simulink model "ControlsWithAutopilot_Properties"  (Simulink 8.4)
settings: Solver=ode45  StartTime=0.0  StopTime=10.0  RelTol=1e-3
undefined symbols (not defined in the file): ap, bias
libraries: simulink x3, discretizing x1
(part 2 of 3)

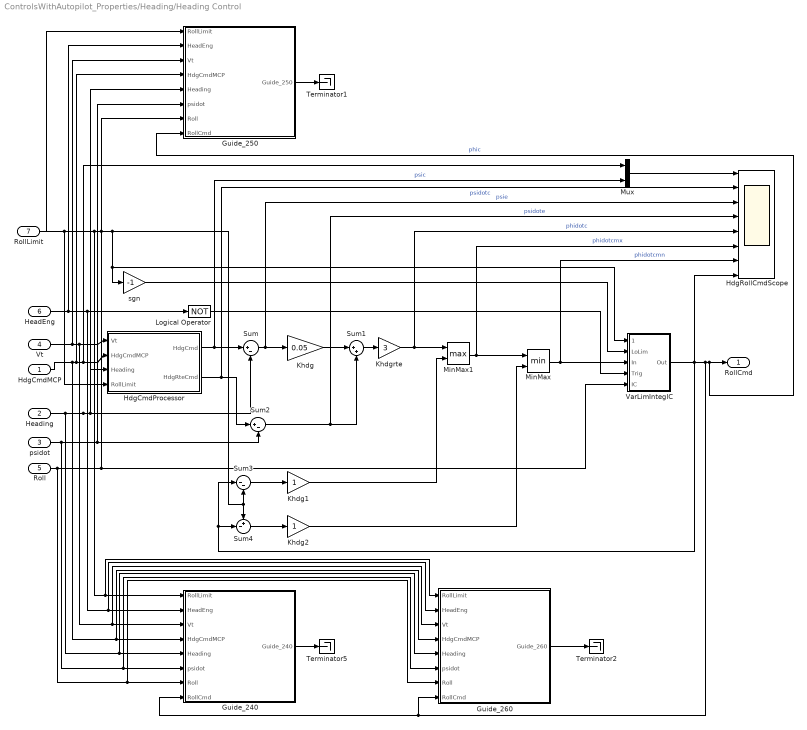
== system ControlsWithAutopilot_Properties/Heading/Heading Control ==
  HdgCmdMCP : Inport  RequirementInfo={} %GIDa_afcd05d1_a9dc_45a7_a8f8_7136ccc61726
  Heading : Inport  RequirementInfo={} %GIDa_19b80fe4_d265_482c_b709_18db80a7cdf3  Port=2
  psidot : Inport  RequirementInfo={} %GIDa_e421e82d_0cc7_4ad7_ac7a_9fb430d189d5  Port=3
  Vt : Inport  RequirementInfo={} %GIDa_9daf3e20_e00e_4f36_b534_d9747a241338  Port=4
  Roll : Inport  RequirementInfo={} %GIDa_8629ba77_a751_4097_af53_617eaa1017be  Port=5
  HeadEng : Inport  RequirementInfo={} %GIDa_dadb1310_2bf4_48cf_8970_85174d784ee3  Port=6
  RollLimit : Inport  Port=7
  Guide_240 : Subsystem  TreatAsAtomicUnit=on  mask(Observer){AnnotationType=ensures, ObserverType=ellipsoid}
      mask prompts: AnnotationType "Type of annotation (pre/post...)"; ObserverType "Observer type"
      mask help:
      | Set an observer for the system.
      | The annotation type parameter sets the type of observer:
      | - requires : pre-condition
      | - ensures : post-condition
      | - assert : an assertion
      | - observer : the observer computes a special type of properties
      mask TypeOptions AnnotationType: ensures | requires | assert | observer
      mask Callback AnnotationType:
      | paramStr = get_param(gcb, 'MaskValues');
      | 
      | if strcmp(paramStr{1}(1),'o')
      |     set_param(gcb,'MaskVisibilities',{'on';'on'});
      |     paramStr{2} = 'ellipsoid';
      |     set_param(gcb,'MaskValues',paramStr);
      | else
      |     set_param(gcb,'MaskVisibilities',{'on';'off'});
      | end
      mask Callback ObserverType:
      | paramStr = get_param(gcb, 'MaskValues');
      | 
      | if strcmp(paramStr{1}(1),'observer')
      |     set_param(gcb,'MaskVisibilities',{'on';'on'});
      |     paramStr{2} = 'ellipsoid';
      |     set_param(gcb,'MaskValues',paramStr);
      | else
      |     set_param(gcb,'MaskVisibilities',{'on';'off'});
      | end
      mask Display:
      | color('red');
      | text(0.5, 0.5, 'Observer Block', 'horizontalAlignment', 'center');
  Guide_250 : Subsystem  TreatAsAtomicUnit=on  mask(Observer){AnnotationType=ensures, ObserverType=ellipsoid}
      mask prompts: AnnotationType "Type of annotation (pre/post...)"; ObserverType "Observer type"
      mask help:
      | Set an observer for the system.
      | The annotation type parameter sets the type of observer:
      | - requires : pre-condition
      | - ensures : post-condition
      | - assert : an assertion
      | - observer : the observer computes a special type of properties
      mask TypeOptions AnnotationType: ensures | requires | assert | observer
      mask Callback AnnotationType:
      | paramStr = get_param(gcb, 'MaskValues');
      | 
      | if strcmp(paramStr{1}(1),'o')
      |     set_param(gcb,'MaskVisibilities',{'on';'on'});
      |     paramStr{2} = 'ellipsoid';
      |     set_param(gcb,'MaskValues',paramStr);
      | else
      |     set_param(gcb,'MaskVisibilities',{'on';'off'});
      | end
      mask Callback ObserverType:
      | paramStr = get_param(gcb, 'MaskValues');
      | 
      | if strcmp(paramStr{1}(1),'observer')
      |     set_param(gcb,'MaskVisibilities',{'on';'on'});
      |     paramStr{2} = 'ellipsoid';
      |     set_param(gcb,'MaskValues',paramStr);
      | else
      |     set_param(gcb,'MaskVisibilities',{'on';'off'});
      | end
      mask Display:
      | color('red');
      | text(0.5, 0.5, 'Observer Block', 'horizontalAlignment', 'center');
  Guide_260 : Subsystem  TreatAsAtomicUnit=on  mask(Observer){AnnotationType=ensures, ObserverType=ellipsoid}
      mask prompts: AnnotationType "Type of annotation (pre/post...)"; ObserverType "Observer type"
      mask help:
      | Set an observer for the system.
      | The annotation type parameter sets the type of observer:
      | - requires : pre-condition
      | - ensures : post-condition
      | - assert : an assertion
      | - observer : the observer computes a special type of properties
      mask TypeOptions AnnotationType: ensures | requires | assert | observer
      mask Callback AnnotationType:
      | paramStr = get_param(gcb, 'MaskValues');
      | 
      | if strcmp(paramStr{1}(1),'o')
      |     set_param(gcb,'MaskVisibilities',{'on';'on'});
      |     paramStr{2} = 'ellipsoid';
      |     set_param(gcb,'MaskValues',paramStr);
      | else
      |     set_param(gcb,'MaskVisibilities',{'on';'off'});
      | end
      mask Callback ObserverType:
      | paramStr = get_param(gcb, 'MaskValues');
      | 
      | if strcmp(paramStr{1}(1),'observer')
      |     set_param(gcb,'MaskVisibilities',{'on';'on'});
      |     paramStr{2} = 'ellipsoid';
      |     set_param(gcb,'MaskValues',paramStr);
      | else
      |     set_param(gcb,'MaskVisibilities',{'on';'off'});
      | end
      mask Display:
      | color('red');
      | text(0.5, 0.5, 'Observer Block', 'horizontalAlignment', 'center');
  HdgCmdProcessor : Subsystem  RequirementInfo={} %GIDa_3cb77e5f_f630_4f22_88a8_7528bfceb83f
  HdgRollCmdScope : Scope  NumInputPorts=8
      settings: RequirementInfo={} %GIDa_5fbe2135_fdf1_4f64_a179_faa1710ae21e  YMin=-30~-30~-10~-10~-4~-10~0~-5  YMax=30~30~10~10~4~10~1~5  SaveName=ScopeData7
  Khdg : Gain  RequirementInfo={} %GIDa_abf81b08_c210_4343_b4da_5a7e229caeb6  Gain=0.05
  Khdg1 : Gain  RequirementInfo={} %GIDa_7a7a35ca_24a5_4d20_bc30_55deea16462c
  Khdg2 : Gain  RequirementInfo={} %GIDa_57191899_7ee5_4454_897a_7009651ed5fb
  Khdgrte : Gain  RequirementInfo={} %GIDa_bcc6a420_18f3_43f0_aaa1_aaa1bbf90f64  Gain=3
  Logical Operator : Logic  RequirementInfo={} %GIDa_5ad405ac_0a88_4b96_aa0e_75483351ee25  Operator=NOT  AllPortsSameDT=off  OutDataTypeStr=boolean
  MinMax : MinMax  RequirementInfo={} %GIDa_4b9381d8_eb85_418b_a975_85846d5ca8c2  Inputs=2
  MinMax1 : MinMax  RequirementInfo={} %GIDa_b40e082d_0fb2_4088_baf4_e9a71be9bcc1  Function=max  Inputs=2
  Mux : Mux  RequirementInfo={} %GIDa_0e83f6c6_ae04_43dd_95fe_a79ec32b40e2  Inputs=2
  Sum : Sum  RequirementInfo={} %GIDa_b89885fc_f86c_4a50_8ce5_47d0488bdc1c  Inputs=|+-
  Sum1 : Sum  RequirementInfo={} %GIDa_40ec6862_b1f8_4f97_ae14_1eadabbceb30  Inputs=|++
  Sum2 : Sum  RequirementInfo={} %GIDa_307d6880_3ab8_4deb_90e0_d68f11d87c85  Inputs=|+-
  Sum3 : Sum  RequirementInfo={} %GIDa_ebb8b765_7f4a_435f_be61_680d3199141b  Inputs=|--
  Sum4 : Sum  RequirementInfo={} %GIDa_05638559_562a_476e_9e4c_91124434a43b  Inputs=+-|
  Terminator1 : Terminator
  Terminator2 : Terminator
  Terminator5 : Terminator
  VarLimIntegIC : Subsystem  RequirementInfo={} %GIDa_7da7eaf5_9731_498e_9aad_b41279918004
  sgn : Gain  RequirementInfo={} %GIDa_84e2dc00_f2e5_41f4_89ce_c9fef234974f  Gain=-1
  RollCmd : Outport  RequirementInfo={} %GIDa_aa862f7f_5d4e_408f_b8c4_26b4ce96fbda
  wires:
  Heading/1 -> Sum/2, HdgCmdProcessor/3(Heading), Guide_250/5(Heading), Guide_240/5(Heading), Guide_260/5(Heading)
  HdgCmdProcessor/1(HdgCmd) -> Sum/1, Mux/2  "psic"
  Sum/1 -> Khdg/1, HdgRollCmdScope/3  "psie"
  Khdg/1 -> Sum1/1
  Sum2/1 -> Sum1/2, HdgRollCmdScope/4  "psidote"
  HdgCmdProcessor/2(HdgRteCmd) -> Sum2/1, HdgRollCmdScope/2  "psidotc"
  psidot/1 -> Sum2/2, Guide_250/6(psidot), Guide_240/6(psidot), Guide_260/6(psidot)
  Vt/1 -> HdgCmdProcessor/1(Vt), Guide_240/3(Vt), Guide_260/3(Vt), Guide_250/3(Vt)
  HdgCmdMCP/1 -> HdgCmdProcessor/2(HdgCmdMCP), Mux/1, Guide_250/4(HdgCmdMCP), Guide_240/4(HdgCmdMCP), Guide_260/4(HdgCmdMCP)
  VarLimIntegIC/1(Out) -> Sum3/1, Sum4/2, HdgRollCmdScope/8, RollCmd/1, Guide_250/8(RollCmd), Guide_240/8(RollCmd), Guide_260/8(RollCmd)  "phic"
  RollLimit/1 -> HdgCmdProcessor/4(RollLimit), Sum4/1, Sum3/2, VarLimIntegIC/1(UpLim), sgn/1, Guide_250/1(RollLimit), Guide_240/1(RollLimit), Guide_260/1(RollLimit)
  sgn/1 -> VarLimIntegIC/2(LoLim)
  Sum1/1 -> Khdgrte/1
  MinMax1/1 -> MinMax/1, HdgRollCmdScope/6  "phidotcmx"
  MinMax/1 -> VarLimIntegIC/3(In), HdgRollCmdScope/7  "phidotcmn"
  HeadEng/1 -> Logical Operator/1, Guide_240/2(HeadEng), Guide_260/2(HeadEng), Guide_250/2(HeadEng)
  Sum3/1 -> Khdg1/1
  Sum4/1 -> Khdg2/1
  Khdg1/1 -> MinMax1/2
  Khdg2/1 -> MinMax/2
  Roll/1 -> VarLimIntegIC/5(IC), Guide_250/7(Roll), Guide_240/7(Roll), Guide_260/7(Roll)
  Khdgrte/1 -> MinMax1/1, HdgRollCmdScope/5  "phidotc"
  Logical Operator/1 -> VarLimIntegIC/4(Trig)
  Mux/1 -> HdgRollCmdScope/1
  Guide_240/1(Guide_240) -> Terminator5/1
  Guide_250/1(Guide_250) -> Terminator1/1
  Guide_260/1(Guide_260) -> Terminator2/1

== system ControlsWithAutopilot_Properties/Heading/ManualOverride ==
  Man : Inport
  Auto : Inport  Port=2
  Switch1 : Switch  RequirementInfo={} %GIDa_5800ea93_45af_42da_974c_4cd975d0b8c8  Criteria=u2 ~= 0  Threshold=0.5
  Out : Outport
  wires:
  Man/1 -> Switch1/3, Switch1/2
  Auto/1 -> Switch1/1
  Switch1/1 -> Out/1

== system ControlsWithAutopilot_Properties/Heading/Roll InnerLoop ==
  note: orig =[0 60 140]
  note: orig = 0.25
  note: orig = 0.8
  RollCmd : Inport  RequirementInfo={} %GIDa_549f9d91_ca5c_4ec7_bf56_cf05f3793396
  Roll : Inport  RequirementInfo={} %GIDa_d885705c_af8c_4e18_b4d1_2f073687ea2c  Port=2
  pdeg : Inport  RequirementInfo={} %GIDa_ba7aa095_15b8_4f85_9051_8b947d28a24d  Port=3
  CAS : Inport  RequirementInfo={} %GIDa_defe4f55_1722_479a_b684_dc07a497c4ef  Port=4
  Kcas_pp : Subsystem  TreatAsAtomicUnit=on
  Kphierr : Gain  RequirementInfo={} %GIDa_96c602a9_a07d_4519_9a2c_04c20a8c958d  Gain=0.5
  Product : Product  RequirementInfo={} %GIDa_6029a1e1_bbec_4e58_a2a6_3f9df62d6e90  RndMeth=Zero
  Roll_IL_scope : Scope  NumInputPorts=7
      settings: RequirementInfo={} %GIDa_ec5ee575_c049_4397_a5dd_5347629f97a6  YMin=-30~-30~-10~-10~-4~-10~0  YMax=30~30~10~10~4~10~1  SaveName=ScopeData5
  Sum : Sum  RequirementInfo={} %GIDa_6dd565f9_cc9c_463a_985b_c182e040d7fd  Inputs=|+-
  Sum1 : Sum  RequirementInfo={} %GIDa_02561aa6_0360_4e6c_b76e_5dde7f2ab3b1  Inputs=|+-
  rollrate_IL : discretizing/Discretized Zero-Pole  RequirementInfo={} %GIDa_636569be_bc7e_4244_84a4_4a62b7fc0808  Zeros=0  Poles=-0.5  Gain=0.00645  AbsTol=auto  SampleTime=1.0  method=zoh  Wc=1
  AilCmd : Outport  RequirementInfo={} %GIDa_cd7ddcd8_c7c7_43e2_be4e_2c0bb3f4c702
  wires:
  Product/1 -> AilCmd/1, Roll_IL_scope/6  "ailcmd"
  Kcas_pp/1(Out) -> Product/2, Roll_IL_scope/7  "kcas"
  Sum1/1 -> Product/1
  CAS/1 -> Kcas_pp/1(In)
  rollrate_IL/1 -> Sum1/2, Roll_IL_scope/5  "pdegwo"
  pdeg/1 -> rollrate_IL/1, Roll_IL_scope/4  "pdeg"
  Kphierr/1 -> Sum1/1
  Roll/1 -> Sum/2, Roll_IL_scope/2  "roll"
  Sum/1 -> Kphierr/1, Roll_IL_scope/3  "rollerr"
  RollCmd/1 -> Sum/1, Roll_IL_scope/1  "rollcmd"

== system ControlsWithAutopilot_Properties/Longitudinal/Altitude Control ==
  engage : Inport  RequirementInfo={} %GIDa_92edc9e2_4cfd_4b16_8fee_8b94964575da
  AltCmd : Inport  RequirementInfo={} %GIDa_edbc7e5c_23e1_4d8f_98c5_e2d77895a510  Port=2
  Altitude : Inport  RequirementInfo={} %GIDa_01b40abf_ece8_4194_aeed_7639b2f9d320  Port=3
  gskts : Inport  RequirementInfo={} %GIDa_49aaf918_ec6b_4cc9_bdad_efb02f39ea3b  Port=4
  hdot : Inport  RequirementInfo={} %GIDa_f8353919_6ca2_40ed_9884_9c34b61b1365  Port=5
  hdotChgRate : Inport  Port=6
  maxHdotChg : Inport  Port=7
  Abs : Abs  RequirementInfo={} %GIDa_1391aa7c_5846_4be5_914e_111d8f2c4215  SaturateOnIntegerOverflow=on
  AltCtnlScope : Scope  NumInputPorts=3
      settings: RequirementInfo={} %GIDa_baad481c_a27b_41ac_bf32_d6e1a7f2cfe1  TimeRange=30  YMin=10000~-5~0  YMax=10200~15~1  SaveName=ScopeData3
  Constant1 : Constant  RequirementInfo={} %GIDa_566c4b52_316f_4d36_82bb_fb65e53f78d2  Value=0
  Divide : Product  RequirementInfo={} %GIDa_b9d1a3fe_7e00_46b2_9426_cf952dcaf391  Inputs=*/
  Kh : Gain  RequirementInfo={} %GIDa_de6b2d53_b3f4_42e2_83e9_439be9ccc299  Gain=0.08
  Logical Operator : Logic  RequirementInfo={} %GIDa_921e6188_0ac2_4a9c_befc_5c7a6835e9e6  Operator=NOT
  Mux : Mux  RequirementInfo={} %GIDa_68aa779e_2c07_4c3b_9ca1_0ecb3161e49a  Inputs=2
  Mux1 : Mux  RequirementInfo={} %GIDa_0a0909f8_d09a_4568_9828_3f29982a74b3  Inputs=2
  Saturation : Saturate  RequirementInfo={} %GIDa_77166b67_e163_40e1_b7e4_7e7410a56d29  UpperLimit=1000  LowerLimit=0.0001
  Sum : Sum  RequirementInfo={} %GIDa_d94a0856_9d8d_4fca_8b77_5f1cf21c0c3a  Inputs=|+-
  Sum3 : Sum  RequirementInfo={} %GIDa_3ee7802b_411f_4586_886f_8bdef6cfccb9  Inputs=|++  SaturateOnIntegerOverflow=on  InputSameDT=on  OutDataTypeStr=Inherit: Same as first input
  Switch : Switch  RequirementInfo={} %GIDa_64af29d5_be60_4de8_bcf5_833ab8e70f35
  Variable  Rate Limit : Subsystem  RequirementInfo={} %GIDa_7d0e1926_4469_4591_916e_2bb88ddee008  TreatAsAtomicUnit=on
  Variable Limit Saturation : Subsystem  RequirementInfo={} %GIDa_0b931211_59c1_4508_94b8_12d4cca2cb6b  TreatAsAtomicUnit=on
  k : Gain  RequirementInfo={} %GIDa_65a0c0b6_6e9b_4a97_b326_1d79079cc625  Gain=-1
  kts2fps : Gain  RequirementInfo={} %GIDa_a49848e7_9841_44de_8ec7_08f1ed28d1e0  Gain=1.6878
  r2d : Gain  RequirementInfo={} %GIDa_934ba914_aaac_471d_9b5e_a120031a3853  Gain=57.2958
  altgamcmd : Outport  RequirementInfo={} %GIDa_3c331913_004d_4e8f_a0a1_b052c80c7670
  wires:
  Sum/1 -> Kh/1
  AltCmd/1 -> Sum/1, Mux/1  "AltCmd"
  Altitude/1 -> Sum/2, Mux/2  "Alt"
  hdot/1 -> Abs/1, Variable  Rate Limit/4(IC)
  Abs/1 -> Sum3/1
  maxHdotChg/1 -> Sum3/2
  k/1 -> Variable Limit Saturation/3(Lo_lim)
  Sum3/1 -> k/1, Variable Limit Saturation/1(up_lim)
  engage/1 -> Switch/2, Logical Operator/1, AltCtnlScope/3  "alteng"
  gskts/1 -> kts2fps/1
  Divide/1 -> r2d/1
  r2d/1 -> altgamcmd/1
  Logical Operator/1 -> Variable  Rate Limit/3(ICtrig)
  Variable Limit Saturation/1(Out1) -> Variable  Rate Limit/2(input), Mux1/1  "hdotc"
  hdotChgRate/1 -> Variable  Rate Limit/1(ratelim)
  Variable  Rate Limit/1(output) -> Divide/1, Mux1/2  "hdotcLim"
  kts2fps/1 -> Saturation/1
  Saturation/1 -> Divide/2
  Switch/1 -> Variable Limit Saturation/2(SigIn)
  Kh/1 -> Switch/1
  Constant1/1 -> Switch/3
  Mux/1 -> AltCtnlScope/1
  Mux1/1 -> AltCtnlScope/2

== system ControlsWithAutopilot_Properties/Longitudinal/EngageORzero ==
  Engage : Inport
  In : Inport  Port=2
  Logical Operator5 : Logic  RequirementInfo={} %GIDa_2faaa958_fdd5_4161_8224_87bc655595ec  AllPortsSameDT=off  OutDataTypeStr=boolean
  Switch1 : Switch  RequirementInfo={} %GIDa_cd8505b1_f38c_41a3_a83c_5e083797b181  Threshold=0.5
  zero10 : Constant  RequirementInfo={} %GIDa_596a5899_ba53_4c37_8272_7211e27ddf24
  zero9 : Constant  RequirementInfo={} %GIDa_b5c8c028_3d9d_45c0_afd9_41cf87627ef7  Value=0
  Out : Outport
  wires:
  Engage/1 -> Logical Operator5/1
  zero10/1 -> Logical Operator5/2
  zero9/1 -> Switch1/3
  In/1 -> Switch1/1
  Logical Operator5/1 -> Switch1/2
  Switch1/1 -> Out/1

== system ControlsWithAutopilot_Properties/Longitudinal/FPA Control ==
  engage : Inport  RequirementInfo={} %GIDa_4330a6b4_8fd7_4be4_8132_0a5a51cb5321
  gamcmd : Inport  RequirementInfo={} %GIDa_72bd14a4_cf4e_4ddf_9979_bc189fd4e864  Port=2
  gamma : Inport  RequirementInfo={} %GIDa_07a290a4_e9be_4e9c_ae2b_d72f5ca4cb2b  Port=3
  thetadeg : Inport  RequirementInfo={} %GIDa_6ddd8d11_1197_4928_a2bc_231a82446ee7  Port=4
  VT : Inport  RequirementInfo={} %GIDa_a0a43ff9_fad6_4fc8_a8cd_c357b3dfb673  Port=5
  FPAScope : Scope  NumInputPorts=4
      settings: RequirementInfo={} %GIDa_08c55925_5efe_4d90_b09d_0072cafa98d7  YMin=-1~-5~-2~-5  YMax=2~5~2~10  SaveName=ScopeData12
  Integ_FPA : DiscreteIntegrator  ExternalReset=level  InitialConditionSource=external  SampleTime=1.0  mask(DiscretizedDiscreteIntegrator){}
      mask init:
      | %zoh
  KIgamerr : Gain  RequirementInfo={} %GIDa_08963e9e_c311_47c8_a63e_11cc7c9fb2d8
  Kgamerr : Gain  RequirementInfo={} %GIDa_3495b1a6_277d_4a6c_aa4f_649fc83b9092  Gain=1.4
  Logical Operator : Logic  RequirementInfo={} %GIDa_eba75fd0_479d_4894_b4e0_0ecea241815c  Operator=NOT  AllPortsSameDT=off  OutDataTypeStr=boolean
  Mux : Mux  RequirementInfo={} %GIDa_ae1e9d70_29ff_4004_97f5_396f2626ff0e  Inputs=2
  Mux1 : Mux  RequirementInfo={} %GIDa_b657458f_9c9c_48b1_af95_f550cfeae5f6  Inputs=2
  Product1 : Product  RequirementInfo={} %GIDa_bb863780_5e58_4e21_8791_e7a2c94dd786  RndMeth=Zero
  Saturation Dynamic : simulink/Discontinuities/Saturation Dynamic  OutMin=[]  OutMax=[]  OutDataTypeStr=Inherit: Same as second input  OutDataType=fixdt(1, 16)  OutScaling=2^-10  DoSatur=off
  Sum : Sum  RequirementInfo={} %GIDa_494c7255_4427_4dad_a3c1_4aee399936eb  Inputs=|++
  Sum1 : Sum  RequirementInfo={} %GIDa_93359946_60e9_438e_99e8_9beddee58b77  Inputs=|+-
  Sum2 : Sum  RequirementInfo={} %GIDa_c5e9feb7_f19d_4066_9b64_2fe045a465c2  Inputs=|+-
  hddLim : Constant  RequirementInfo={} %GIDa_1bf124ef_f3a0_4770_a704_52ef6436d4b5  Value=4.83*57.2958
  kt2fps : Gain  RequirementInfo={} %GIDa_c7ee5a6f_140d_48a3_b5c5_8ced7bef0603  Gain=1.6878
  m1 : Gain  RequirementInfo={} %GIDa_3e310fb8_58d1_4ad2_a1bc_b1914379a108  Gain=-1
  PitchCmd : Outport  RequirementInfo={} %GIDa_7e56bb7b_bd21_4466_8889_6a6d9858a2da
  wires:
  Sum1/1 -> PitchCmd/1, FPAScope/4  "PitchCmd"
  Kgamerr/1 -> Sum1/2, Sum/2
  Integ_FPA/1 -> Sum1/1
  gamma/1 -> Kgamerr/1, Sum2/2, Mux/2  "gamma"
  thetadeg/1 -> Sum/1
  Sum/1 -> Integ_FPA/3
  engage/1 -> Logical Operator/1, FPAScope/1  "engage"
  Logical Operator/1 -> Integ_FPA/2
  kt2fps/1 -> Product1/2
  hddLim/1 -> Product1/1
  Product1/1 -> Saturation Dynamic/1, m1/1
  VT/1 -> kt2fps/1
  Saturation Dynamic/1 -> Integ_FPA/1, Mux1/2  "gamerrlim"
  KIgamerr/1 -> Saturation Dynamic/2
  m1/1 -> Saturation Dynamic/3
  Sum2/1 -> KIgamerr/1, Mux1/1  "gamerr"
  gamcmd/1 -> Sum2/1, Mux/1  "gamcmd"
  Mux/1 -> FPAScope/2
  Mux1/1 -> FPAScope/3

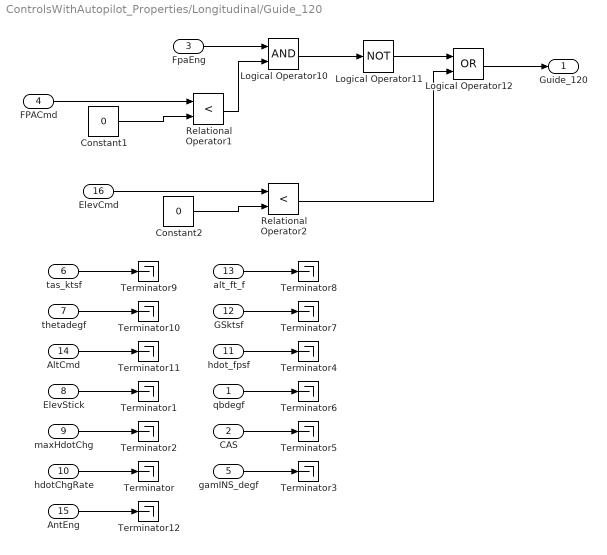
== system ControlsWithAutopilot_Properties/Longitudinal/Guide_120 ==
  qbdegf : Inport
  CAS : Inport  Port=2
  FpaEng : Inport  Port=3
  FPACmd : Inport  Port=4
  gamINS_degf : Inport  Port=5
  tas_ktsf : Inport  Port=6
  thetadegf : Inport  Port=7
  ElevStick : Inport  Port=8
  maxHdotChg : Inport  Port=9
  hdotChgRate : Inport  Port=10
  hdot_fpsf : Inport  Port=11
  GSktsf : Inport  Port=12
  alt_ft_f : Inport  Port=13
  AltCmd : Inport  Port=14
  AntEng : Inport  Port=15
  ElevCmd : Inport  Port=16
  Constant1 : Constant  Value=0
  Constant2 : Constant  Value=0
  Logical Operator10 : Logic  AllPortsSameDT=off  OutDataTypeStr=boolean
  Logical Operator11 : Logic  Operator=NOT  AllPortsSameDT=off  OutDataTypeStr=boolean
  Logical Operator12 : Logic  Operator=OR  AllPortsSameDT=off  OutDataTypeStr=boolean
  Relational Operator1 : RelationalOperator  Operator=<  OutDataTypeStr=boolean
  Relational Operator2 : RelationalOperator  Operator=<  OutDataTypeStr=boolean
  Terminator{,1..12} (13 alike) : Terminator
  Guide_120 : Outport
  wires:
  hdotChgRate/1 -> Terminator/1
  maxHdotChg/1 -> Terminator2/1
  ElevStick/1 -> Terminator1/1
  CAS/1 -> Terminator5/1
  qbdegf/1 -> Terminator6/1
  Constant2/1 -> Relational Operator2/2
  ElevCmd/1 -> Relational Operator2/1
  FpaEng/1 -> Logical Operator10/1
  Constant1/1 -> Relational Operator1/2
  FPACmd/1 -> Relational Operator1/1
  Relational Operator1/1 -> Logical Operator10/2
  Logical Operator11/1 -> Logical Operator12/1
  Logical Operator10/1 -> Logical Operator11/1
  Relational Operator2/1 -> Logical Operator12/2
  Logical Operator12/1 -> Guide_120/1
  alt_ft_f/1 -> Terminator8/1
  GSktsf/1 -> Terminator7/1
  hdot_fpsf/1 -> Terminator4/1
  gamINS_degf/1 -> Terminator3/1
  tas_ktsf/1 -> Terminator9/1
  thetadegf/1 -> Terminator10/1
  AltCmd/1 -> Terminator11/1
  AntEng/1 -> Terminator12/1

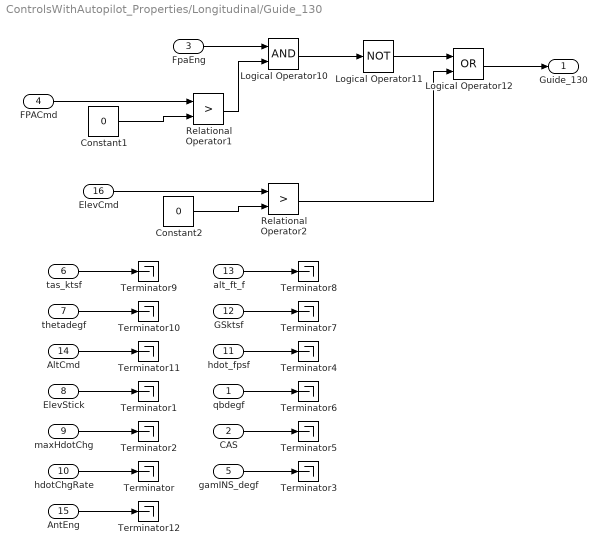
== system ControlsWithAutopilot_Properties/Longitudinal/Guide_130 ==
  qbdegf : Inport
  CAS : Inport  Port=2
  FpaEng : Inport  Port=3
  FPACmd : Inport  Port=4
  gamINS_degf : Inport  Port=5
  tas_ktsf : Inport  Port=6
  thetadegf : Inport  Port=7
  ElevStick : Inport  Port=8
  maxHdotChg : Inport  Port=9
  hdotChgRate : Inport  Port=10
  hdot_fpsf : Inport  Port=11
  GSktsf : Inport  Port=12
  alt_ft_f : Inport  Port=13
  AltCmd : Inport  Port=14
  AntEng : Inport  Port=15
  ElevCmd : Inport  Port=16
  Constant1 : Constant  Value=0
  Constant2 : Constant  Value=0
  Logical Operator10 : Logic  AllPortsSameDT=off  OutDataTypeStr=boolean
  Logical Operator11 : Logic  Operator=NOT  AllPortsSameDT=off  OutDataTypeStr=boolean
  Logical Operator12 : Logic  Operator=OR  AllPortsSameDT=off  OutDataTypeStr=boolean
  Relational Operator1 : RelationalOperator  Operator=>  OutDataTypeStr=boolean
  Relational Operator2 : RelationalOperator  Operator=>  OutDataTypeStr=boolean
  Terminator{,1..12} (13 alike) : Terminator
  Guide_130 : Outport
  wires:
  hdotChgRate/1 -> Terminator/1
  maxHdotChg/1 -> Terminator2/1
  ElevStick/1 -> Terminator1/1
  CAS/1 -> Terminator5/1
  qbdegf/1 -> Terminator6/1
  Constant2/1 -> Relational Operator2/2
  ElevCmd/1 -> Relational Operator2/1
  FpaEng/1 -> Logical Operator10/1
  Constant1/1 -> Relational Operator1/2
  FPACmd/1 -> Relational Operator1/1
  Relational Operator1/1 -> Logical Operator10/2
  Logical Operator11/1 -> Logical Operator12/1
  Logical Operator10/1 -> Logical Operator11/1
  Relational Operator2/1 -> Logical Operator12/2
  Logical Operator12/1 -> Guide_130/1
  alt_ft_f/1 -> Terminator8/1
  GSktsf/1 -> Terminator7/1
  hdot_fpsf/1 -> Terminator4/1
  gamINS_degf/1 -> Terminator3/1
  tas_ktsf/1 -> Terminator9/1
  thetadegf/1 -> Terminator10/1
  AltCmd/1 -> Terminator11/1
  AntEng/1 -> Terminator12/1

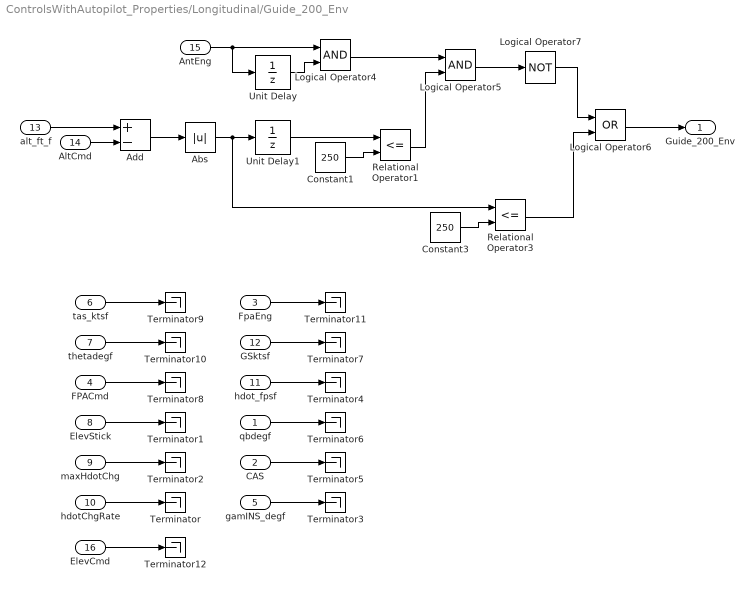
== system ControlsWithAutopilot_Properties/Longitudinal/Guide_200_Env ==
  qbdegf : Inport
  CAS : Inport  Port=2
  FpaEng : Inport  Port=3
  FPACmd : Inport  Port=4
  gamINS_degf : Inport  Port=5
  tas_ktsf : Inport  Port=6
  thetadegf : Inport  Port=7
  ElevStick : Inport  Port=8
  maxHdotChg : Inport  Port=9
  hdotChgRate : Inport  Port=10
  hdot_fpsf : Inport  Port=11
  GSktsf : Inport  Port=12
  alt_ft_f : Inport  Port=13
  AltCmd : Inport  Port=14
  AntEng : Inport  Port=15
  ElevCmd : Inport  Port=16
  Abs : Abs
  Add : Sum  Inputs=+-
  Constant1 : Constant  Value=250
  Constant3 : Constant  Value=250
  Logical Operator4 : Logic  AllPortsSameDT=off  OutDataTypeStr=boolean
  Logical Operator5 : Logic  AllPortsSameDT=off  OutDataTypeStr=boolean
  Logical Operator6 : Logic  Operator=OR  AllPortsSameDT=off  OutDataTypeStr=boolean
  Logical Operator7 : Logic  Operator=NOT  AllPortsSameDT=off  OutDataTypeStr=boolean
  Relational Operator1 : RelationalOperator  Operator=<=  OutDataTypeStr=boolean
  Relational Operator3 : RelationalOperator  Operator=<=  OutDataTypeStr=boolean
  Terminator{,1..12} (13 alike) : Terminator
  Unit Delay : UnitDelay  SampleTime=-1
  Unit Delay1 : UnitDelay  SampleTime=-1
  Guide_200_Env : Outport
  wires:
  hdotChgRate/1 -> Terminator/1
  maxHdotChg/1 -> Terminator2/1
  ElevStick/1 -> Terminator1/1
  CAS/1 -> Terminator5/1
  qbdegf/1 -> Terminator6/1
  GSktsf/1 -> Terminator7/1
  hdot_fpsf/1 -> Terminator4/1
  gamINS_degf/1 -> Terminator3/1
  tas_ktsf/1 -> Terminator9/1
  thetadegf/1 -> Terminator10/1
  FpaEng/1 -> Terminator11/1
  FPACmd/1 -> Terminator8/1
  ElevCmd/1 -> Terminator12/1
  AntEng/1 -> Unit Delay/1, Logical Operator4/1
  Unit Delay/1 -> Logical Operator4/2
  Logical Operator4/1 -> Logical Operator5/1
  Add/1 -> Abs/1
  AltCmd/1 -> Add/2
  alt_ft_f/1 -> Add/1
  Abs/1 -> Relational Operator3/1, Unit Delay1/1
  Constant1/1 -> Relational Operator1/2
  Unit Delay1/1 -> Relational Operator1/1
  Relational Operator1/1 -> Logical Operator5/2
  Logical Operator7/1 -> Logical Operator6/1
  Logical Operator5/1 -> Logical Operator7/1
  Constant3/1 -> Relational Operator3/2
  Relational Operator3/1 -> Logical Operator6/2
  Logical Operator6/1 -> Guide_200_Env/1

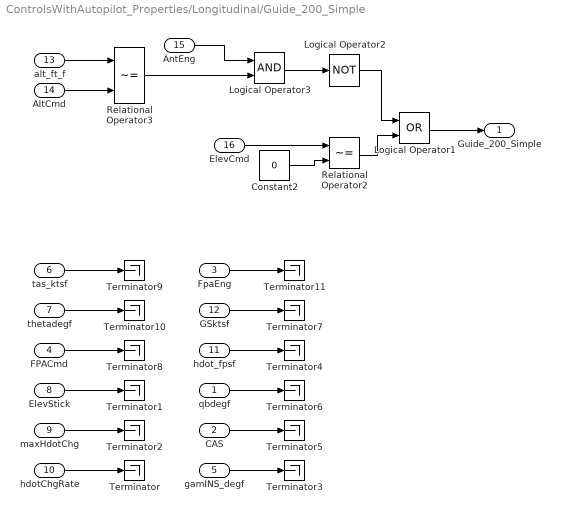
== system ControlsWithAutopilot_Properties/Longitudinal/Guide_200_Simple ==
  qbdegf : Inport
  CAS : Inport  Port=2
  FpaEng : Inport  Port=3
  FPACmd : Inport  Port=4
  gamINS_degf : Inport  Port=5
  tas_ktsf : Inport  Port=6
  thetadegf : Inport  Port=7
  ElevStick : Inport  Port=8
  maxHdotChg : Inport  Port=9
  hdotChgRate : Inport  Port=10
  hdot_fpsf : Inport  Port=11
  GSktsf : Inport  Port=12
  alt_ft_f : Inport  Port=13
  AltCmd : Inport  Port=14
  AntEng : Inport  Port=15
  ElevCmd : Inport  Port=16
  Constant2 : Constant  Value=0
  Logical Operator1 : Logic  Operator=OR  AllPortsSameDT=off  OutDataTypeStr=boolean
  Logical Operator2 : Logic  Operator=NOT  AllPortsSameDT=off  OutDataTypeStr=boolean
  Logical Operator3 : Logic  AllPortsSameDT=off  OutDataTypeStr=boolean
  Relational Operator2 : RelationalOperator  Operator=~=  OutDataTypeStr=boolean
  Relational Operator3 : RelationalOperator  Operator=~=  OutDataTypeStr=boolean
  Terminator{,1..11} (12 alike) : Terminator
  Guide_200_Simple : Outport
  wires:
  hdotChgRate/1 -> Terminator/1
  maxHdotChg/1 -> Terminator2/1
  ElevStick/1 -> Terminator1/1
  CAS/1 -> Terminator5/1
  qbdegf/1 -> Terminator6/1
  GSktsf/1 -> Terminator7/1
  hdot_fpsf/1 -> Terminator4/1
  gamINS_degf/1 -> Terminator3/1
  tas_ktsf/1 -> Terminator9/1
  thetadegf/1 -> Terminator10/1
  Constant2/1 -> Relational Operator2/2
  ElevCmd/1 -> Relational Operator2/1
  Relational Operator2/1 -> Logical Operator1/2
  Logical Operator2/1 -> Logical Operator1/1
  Logical Operator1/1 -> Guide_200_Simple/1
  AntEng/1 -> Logical Operator3/1
  alt_ft_f/1 -> Relational Operator3/1
  AltCmd/1 -> Relational Operator3/2
  Relational Operator3/1 -> Logical Operator3/2
  Logical Operator3/1 -> Logical Operator2/1
  FpaEng/1 -> Terminator11/1
  FPACmd/1 -> Terminator8/1

== system ControlsWithAutopilot_Properties/Longitudinal/ManualOverride ==
  Man : Inport
  Auto : Inport  Port=2
  Switch1 : Switch  RequirementInfo={} %GIDa_891c72b6_c029_43c0_848a_219761f8f015  Criteria=u2 ~= 0  Threshold=0.5
  Out : Outport
  wires:
  Man/1 -> Switch1/3, Switch1/2
  Auto/1 -> Switch1/1
  Switch1/1 -> Out/1

== system ControlsWithAutopilot_Properties/Longitudinal/Pitch InnerLoop ==
  PitchCmd : Inport  RequirementInfo={} %GIDa_e681796d_a620_4c95_b4ed_ba3232dc70a2
  Pitch : Inport  RequirementInfo={} %GIDa_6f4baf24_a090_49e6_89b2_2ff3bd4fd377  Port=2
  qdeg : Inport  RequirementInfo={} %GIDa_13210493_e26c_4a14_89fc_8ad0299ca616  Port=3
  CAS : Inport  RequirementInfo={} %GIDa_e1a07f62_5dbf_46dc_bc2c_c2998ea01de8  Port=4
  Kcas_pp : Subsystem  TreatAsAtomicUnit=on
  Kpitch : Gain  RequirementInfo={} %GIDa_4a392bdb_3184_422c_b598_a156d3e8b02c  Gain=2
  Kwo : Gain  RequirementInfo={} %GIDa_6174b3c5_b132_42d6_a380_7a86f841c8e6  Gain=0.5
  Mux : Mux  RequirementInfo={} %GIDa_93279ee0_cc4a_4a25_b0b1_b731353743b0  Inputs=2
  PitchScope : Scope  NumInputPorts=6
      settings: RequirementInfo={} %GIDa_5646223d_16bd_44bf_9f51_c97977b5f9c0  YMin=-2~-2~-2~-20~-20~0  YMax=10~2~2~20~20~1.2  SaveName=ScopeData11
  Product : Product  RequirementInfo={} %GIDa_ee2099f1_df06_4fc6_bf9b_0b7652de3a20  RndMeth=Zero
  Sum : Sum  RequirementInfo={} %GIDa_6e966264_2a04_4ed3_91bc_90c4039fd9a0  Inputs=|+-
  Sum1 : Sum  RequirementInfo={} %GIDa_5254d09e_07d7_42ec_bb70_93117997e359  Inputs=|-+
  Transfer Fcn_pp : Subsystem  TreatAsAtomicUnit=on
  ElevCmd : Outport  RequirementInfo={} %GIDa_133d9978_a863_4cc3_b149_7ebb5beb5068
  wires:
  Sum/1 -> Kpitch/1, PitchScope/2  "Pitcherror"
  Pitch/1 -> Sum/2, Mux/2
  Kpitch/1 -> Sum1/1
  qdeg/1 -> Transfer Fcn_pp/1(Inport1)
  Transfer Fcn_pp/1(Outport1) -> Kwo/1
  CAS/1 -> Kcas_pp/1(In)
  Sum1/1 -> Product/1, PitchScope/4  "dec"
  Kcas_pp/1(Out) -> Product/2, PitchScope/6  "Kcas"
  Product/1 -> ElevCmd/1, PitchScope/5  "elevcmd"
  Kwo/1 -> Sum1/2, PitchScope/3  "qdegwo"
  PitchCmd/1 -> Sum/1, Mux/1  "Pitchcmd"
  Mux/1 -> PitchScope/1

== system ControlsWithAutopilot_Properties/Yaw Damper/EngageORzero ==
  Engage : Inport
  In : Inport  Port=2
  Logical Operator5 : Logic  RequirementInfo={} %GIDa_039f8944_4af0_4d9a_b296_dc63f4fb9b24  AllPortsSameDT=off  OutDataTypeStr=boolean
  Switch1 : Switch  RequirementInfo={} %GIDa_5a57b0db_bac7_4f14_9c86_f79c8d73773a  Threshold=0.5
  zero10 : Constant  RequirementInfo={} %GIDa_459066bd_0987_4218_99ad_2fd246291f08
  zero9 : Constant  RequirementInfo={} %GIDa_11be025e_2612_434d_af1e_162a733bf0cc  Value=0
  Out : Outport
  wires:
  Engage/1 -> Logical Operator5/1
  zero10/1 -> Logical Operator5/2
  zero9/1 -> Switch1/3
  In/1 -> Switch1/1
  Logical Operator5/1 -> Switch1/2
  Switch1/1 -> Out/1

== system ControlsWithAutopilot_Properties/Yaw Damper/Kcas_pp ==
  In : Inport
  CompInfEq2 : RelationalOperator  Operator=<=  InputSameDT=on
  CompInfEq3 : RelationalOperator  Operator=<=  InputSameDT=on
  CompInfEq4 : RelationalOperator  Operator=<=  InputSameDT=on
  CompSup1 : RelationalOperator  InputSameDT=on
  CompSup2 : RelationalOperator  Operator=>  InputSameDT=on
  CompSup3 : RelationalOperator  Operator=>  InputSameDT=on
  Data1 : Constant
  Data2 : Constant
  Data3 : Constant  Value=0.3
  Data4 : Constant  Value=0.3
  Idx1 : Constant  Value=0
  Idx2 : Constant  Value=120
  Idx3 : Constant  Value=350
  Idx4 : Constant  Value=500
  Interpolate1 : Subsystem
  Interpolate2 : Subsystem
  Interpolate3 : Subsystem
  Product1 : Product  Inputs=***  SaturateOnIntegerOverflow=on  RndMeth=Zero  OutDataTypeStr=Inherit: Same as first input
  Product2 : Product  Inputs=***  SaturateOnIntegerOverflow=on  RndMeth=Zero  OutDataTypeStr=Inherit: Same as first input
  Product3 : Product  Inputs=***  SaturateOnIntegerOverflow=on  RndMeth=Zero  OutDataTypeStr=Inherit: Same as first input
  Sum : Sum  Inputs=+++  SaturateOnIntegerOverflow=on  InputSameDT=on  OutDataTypeStr=Inherit: Same as first input
  Out : Outport
  wires:
  In/1 -> Interpolate1/1(InportIn), CompSup1/1, Interpolate2/1(InportIn), CompSup2/1, CompInfEq2/1, Interpolate3/1(InportIn), CompSup3/1, CompInfEq3/1, CompInfEq4/1
  Idx1/1 -> Interpolate1/2(InportIdx1), CompSup1/2
  Data1/1 -> Interpolate1/4(InportData1)
  Interpolate1/1(Out) -> Product1/1
  CompSup1/1 -> Product1/2
  CompInfEq2/1 -> Product1/3
  Product1/1 -> Sum/1
  Idx2/1 -> Interpolate2/2(InportIdx1), CompSup2/2, Interpolate1/3(InportIdx2), CompInfEq2/2
  Data2/1 -> Interpolate2/4(InportData1), Interpolate1/5(InportData2)
  Interpolate2/1(Out) -> Product2/1
  CompSup2/1 -> Product2/2
  CompInfEq3/1 -> Product2/3
  Product2/1 -> Sum/2
  Idx3/1 -> Interpolate3/2(InportIdx1), CompSup3/2, Interpolate2/3(InportIdx2), CompInfEq3/2
  Data3/1 -> Interpolate3/4(InportData1), Interpolate2/5(InportData2)
  Interpolate3/1(Out) -> Product3/1
  CompSup3/1 -> Product3/2
  CompInfEq4/1 -> Product3/3
  Product3/1 -> Sum/3
  Idx4/1 -> Interpolate3/3(InportIdx2), CompInfEq4/2
  Data4/1 -> Interpolate3/5(InportData2)
  Sum/1 -> Out/1

== system ControlsWithAutopilot_Properties/Yaw Damper/ManualOverride ==
  Man : Inport
  Auto : Inport  Port=2
  Switch1 : Switch  RequirementInfo={} %GIDa_c20200e4_a463_47a4_8bca_86ae3712d2e3  Criteria=u2 ~= 0  Threshold=0.5
  Out : Outport
  wires:
  Man/1 -> Switch1/3, Switch1/2
  Auto/1 -> Switch1/1
  Switch1/1 -> Out/1

== system ControlsWithAutopilot_Properties/Yaw Damper/YD_wo_pp ==
  Inport1 : Inport
  D1 : UnitDelay  SampleTime=-1
  GainAC1_1 : Gain  Gain=-10  SaturateOnIntegerOverflow=on  OutDataTypeStr=Inherit: Same as input  ParamDataTypeStr=Inherit: Same as input
  GainAC2_1 : Gain  Gain=-10  SaturateOnIntegerOverflow=on  OutDataTypeStr=Inherit: Same as input  ParamDataTypeStr=Inherit: Same as input
  GainBD1_1 : Gain  SaturateOnIntegerOverflow=on  OutDataTypeStr=Inherit: Same as input  ParamDataTypeStr=Inherit: Same as input
  GainBD2_1 : Gain  SaturateOnIntegerOverflow=on  OutDataTypeStr=Inherit: Same as input  ParamDataTypeStr=Inherit: Same as input
  Sum1 : Sum  SaturateOnIntegerOverflow=on  InputSameDT=on  OutDataTypeStr=Inherit: Same as first input
  Sum2 : Sum  SaturateOnIntegerOverflow=on  InputSameDT=on  OutDataTypeStr=Inherit: Same as first input
  Outport1 : Outport
  wires:
  D1/1 -> GainAC1_1/1, GainAC2_1/1
  GainAC1_1/1 -> Sum1/1
  GainAC2_1/1 -> Sum2/1
  Inport1/1 -> GainBD1_1/1, GainBD2_1/1
  GainBD1_1/1 -> Sum1/2
  GainBD2_1/1 -> Sum2/2
  Sum1/1 -> D1/1
  Sum2/1 -> Outport1/1

== system ControlsWithAutopilot_Properties/Heading/Heading Control/Guide_240 ==
  RollLimit : Inport
  HeadEng : Inport  Port=2
  Vt : Inport  Port=3
  HdgCmdMCP : Inport  Port=4
  Heading : Inport  Port=5
  psidot : Inport  Port=6
  Roll : Inport  Port=7
  RollCmd : Inport  Port=8
  Abs : Abs
  Relational Operator : RelationalOperator  Operator=<  OutDataTypeStr=boolean
  Terminator{,1..5} (6 alike) : Terminator
  Guide_240 : Outport
  wires:
  Roll/1 -> Terminator/1
  HeadEng/1 -> Terminator5/1
  Vt/1 -> Terminator4/1
  HdgCmdMCP/1 -> Terminator3/1
  Heading/1 -> Terminator2/1
  psidot/1 -> Terminator1/1
  RollCmd/1 -> Abs/1
  Abs/1 -> Relational Operator/1
  RollLimit/1 -> Relational Operator/2
  Relational Operator/1 -> Guide_240/1

== system ControlsWithAutopilot_Properties/Heading/Heading Control/Guide_250 ==
  RollLimit : Inport
  HeadEng : Inport  Port=2
  Vt : Inport  Port=3
  HdgCmdMCP : Inport  Port=4
  Heading : Inport  Port=5
  psidot : Inport  Port=6
  Roll : Inport  Port=7
  RollCmd : Inport  Port=8
  Constant : Constant  Value=0
  Logical Operator : Logic  Operator=XOR  AllPortsSameDT=off  OutDataTypeStr=boolean
  Logical Operator1 : Logic  Operator=NOT  AllPortsSameDT=off  OutDataTypeStr=boolean
  Logical Operator2 : Logic  Operator=OR  AllPortsSameDT=off  OutDataTypeStr=boolean
  Logical Operator3 : Logic  Operator=NOT  AllPortsSameDT=off  OutDataTypeStr=boolean
  Relational Operator : RelationalOperator  Operator===  OutDataTypeStr=boolean
  Relational Operator2 : RelationalOperator  Operator===  OutDataTypeStr=boolean
  Terminator{,1..2,4} (4 alike) : Terminator
  Guide_250 : Outport
  wires:
  Roll/1 -> Terminator/1
  Vt/1 -> Terminator4/1
  psidot/1 -> Terminator1/1
  RollLimit/1 -> Terminator2/1
  Heading/1 -> Relational Operator/1
  HdgCmdMCP/1 -> Relational Operator/2
  RollCmd/1 -> Relational Operator2/1
  Constant/1 -> Relational Operator2/2
  Relational Operator2/1 -> Logical Operator/1
  Relational Operator/1 -> Logical Operator/2
  Logical Operator/1 -> Logical Operator1/1
  HeadEng/1 -> Logical Operator3/1
  Logical Operator1/1 -> Logical Operator2/1
  Logical Operator3/1 -> Logical Operator2/2
  Logical Operator2/1 -> Guide_250/1

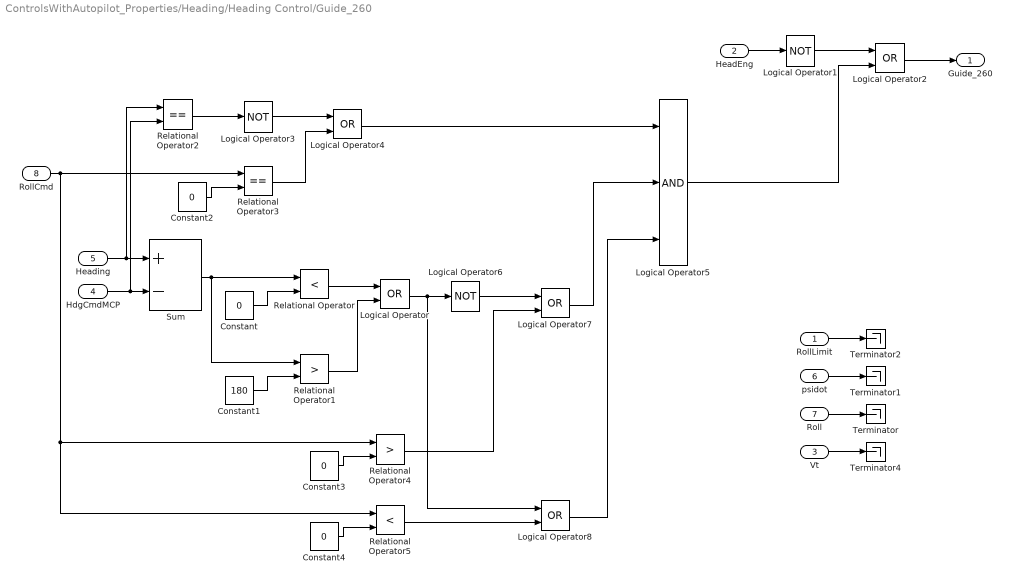
== system ControlsWithAutopilot_Properties/Heading/Heading Control/Guide_260 ==
  RollLimit : Inport
  HeadEng : Inport  Port=2
  Vt : Inport  Port=3
  HdgCmdMCP : Inport  Port=4
  Heading : Inport  Port=5
  psidot : Inport  Port=6
  Roll : Inport  Port=7
  RollCmd : Inport  Port=8
  Constant{,2..4} (4 alike) : Constant  Value=0
  Constant1 : Constant  Value=180
  Logical Operator{,2,4,7..8} (5 alike) : Logic  Operator=OR  AllPortsSameDT=off  OutDataTypeStr=boolean
  Logical Operator1 : Logic  Operator=NOT  AllPortsSameDT=off  OutDataTypeStr=boolean
  Logical Operator3 : Logic  Operator=NOT  AllPortsSameDT=off  OutDataTypeStr=boolean
  Logical Operator5 : Logic  Inputs=3  AllPortsSameDT=off  OutDataTypeStr=boolean
  Logical Operator6 : Logic  Operator=NOT  AllPortsSameDT=off  OutDataTypeStr=boolean
  Relational Operator : RelationalOperator  Operator=<  OutDataTypeStr=boolean
  Relational Operator1 : RelationalOperator  Operator=>  OutDataTypeStr=boolean
  Relational Operator2 : RelationalOperator  Operator===  OutDataTypeStr=boolean
  Relational Operator3 : RelationalOperator  Operator===  OutDataTypeStr=boolean
  Relational Operator4 : RelationalOperator  Operator=>  OutDataTypeStr=boolean
  Relational Operator5 : RelationalOperator  Operator=<  OutDataTypeStr=boolean
  Sum : Sum  Inputs=+-
  Terminator{,1..2,4} (4 alike) : Terminator
  Guide_260 : Outport
  wires:
  Roll/1 -> Terminator/1
  Vt/1 -> Terminator4/1
  psidot/1 -> Terminator1/1
  RollLimit/1 -> Terminator2/1
  Heading/1 -> Sum/1, Relational Operator2/1
  HdgCmdMCP/1 -> Sum/2, Relational Operator2/2
  Sum/1 -> Relational Operator/1, Relational Operator1/1
  Constant/1 -> Relational Operator/2
  Relational Operator/1 -> Logical Operator/1
  Constant1/1 -> Relational Operator1/2
  Relational Operator1/1 -> Logical Operator/2
  HeadEng/1 -> Logical Operator1/1
  Logical Operator1/1 -> Logical Operator2/1
  Logical Operator2/1 -> Guide_260/1
  Logical Operator3/1 -> Logical Operator4/1
  Relational Operator2/1 -> Logical Operator3/1
  RollCmd/1 -> Relational Operator3/1, Relational Operator4/1, Relational Operator5/1
  Constant2/1 -> Relational Operator3/2
  Relational Operator3/1 -> Logical Operator4/2
  Logical Operator4/1 -> Logical Operator5/1
  Constant3/1 -> Relational Operator4/2
  Logical Operator/1 -> Logical Operator6/1, Logical Operator8/1
  Logical Operator6/1 -> Logical Operator7/1
  Relational Operator4/1 -> Logical Operator7/2
  Logical Operator7/1 -> Logical Operator5/2
  Constant4/1 -> Relational Operator5/2
  Relational Operator5/1 -> Logical Operator8/2
  Logical Operator8/1 -> Logical Operator5/3
  Logical Operator5/1 -> Logical Operator2/2

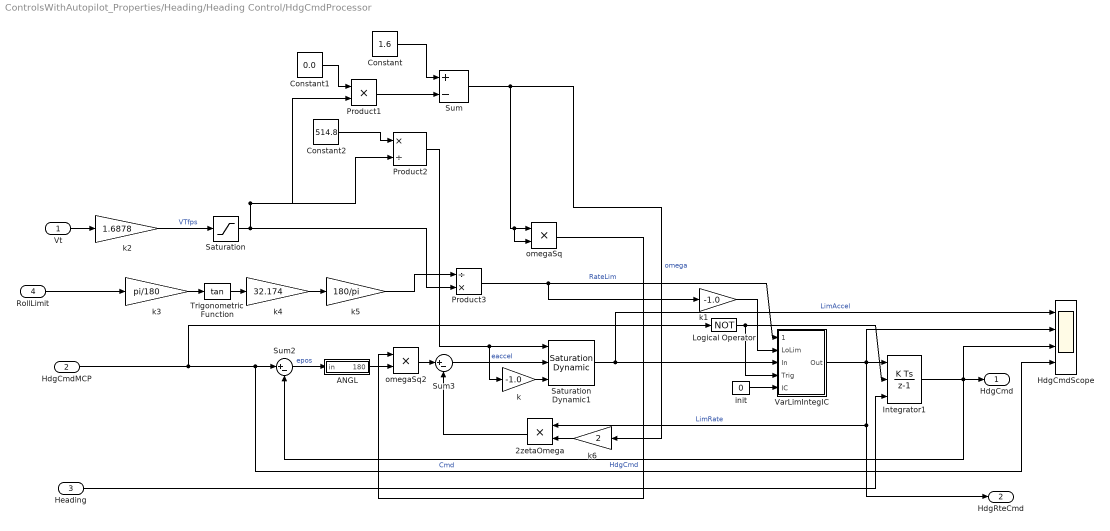
== system ControlsWithAutopilot_Properties/Heading/Heading Control/HdgCmdProcessor ==
  Vt : Inport  RequirementInfo={} %GIDa_aea371ad_7692_43c3_9333_237397a7088d
  HdgCmdMCP : Inport  RequirementInfo={} %GIDa_62146feb_aace_4fc2_8116_9e6cd7e3722f  Port=2
  Heading : Inport  RequirementInfo={} %GIDa_2367d888_2282_4a9b_9dc0_ce749bdb20fa  Port=3
  RollLimit : Inport  Port=4
  2zetaOmega : Product  RequirementInfo={} %GIDa_f321de1d_2313_4525_97dc_b8d5cf0673a7  RndMeth=Zero
  ANGL : Subsystem  RequirementInfo={} %GIDa_a65114d8_8cfa_43a6_b93e_efba84d5b466
  Constant : Constant  Value=1.6
  Constant1 : Constant  Value=0.0
  Constant2 : Constant  Value=514.8
  HdgCmdScope : Scope  NumInputPorts=4
      settings: RequirementInfo={} %GIDa_44f9dfb2_1047_4c85_9993_6df91b14ae0d  YMin=-2~-4~-40~-40  YMax=2~4~40~40  SaveName=ScopeData6
  Integrator1 : DiscreteIntegrator  ExternalReset=level  InitialConditionSource=external  SampleTime=1.0  mask(DiscretizedDiscreteIntegrator){}
      mask init:
      | %zoh
  Logical Operator : Logic  RequirementInfo={} %GIDa_a3be1b8e_7e30_4ddb_8576_d6096a49c77e  Operator=NOT  AllPortsSameDT=off  OutDataTypeStr=boolean
  Product1 : Product  RndMeth=Zero
  Product2 : Product  Inputs=*/  RndMeth=Zero
  Product3 : Product  Inputs=/*  RndMeth=Zero
  Saturation : Saturate  RequirementInfo={} %GIDa_34361c95_77fe_4878_a89a_f2e2245d083f  UpperLimit=1000  LowerLimit=0.0001
  Saturation Dynamic1 : simulink/Discontinuities/Saturation Dynamic  RequirementInfo={} %GIDa_3c1bb0e4_035b_467b_b908_73d0679fa8c4  OutMin=[]  OutMax=[]  OutDataTypeStr=Inherit: Same as second input  OutDataType=fixdt(1, 16)  OutScaling=2^-10  DoSatur=off
  Sum : Sum  Inputs=+-
  Sum2 : Sum  RequirementInfo={} %GIDa_0134b7ed_8c9c_449a_ac58_c6bc449e5dc3  Inputs=|+-
  Sum3 : Sum  RequirementInfo={} %GIDa_133a47a4_a1d1_45cf_bb65_a8e707312c61  Inputs=|+-
  Trigonometric Function : Trigonometry  RequirementInfo={} %GIDa_9fedb248_844e_457e_a851_4a39016fb810  Operator=tan
  VarLimIntegIC : Subsystem  RequirementInfo={} %GIDa_5e236912_7c4b_441a_a6c7_d31391da156a
  init : Constant  RequirementInfo={} %GIDa_bb6a6882_f5a4_4f54_8f02_3d74a10327cc  Value=0
  k : Gain  RequirementInfo={} %GIDa_b3adcecb_db12_4f0e_a73c_fd191106ac98  Gain=-1.0
  k1 : Gain  RequirementInfo={} %GIDa_4080639b_e5dd_4b50_81e0_40e346cb6275  Gain=-1.0
  k2 : Gain  RequirementInfo={} %GIDa_3129ff2a_7a94_46f5_a52d_bf604afbaa9d  Gain=1.6878
  k3 : Gain  RequirementInfo={} %GIDa_bc42355c_264a_47e1_8506_c4c4e8e068fc  Gain=pi/180
  k4 : Gain  RequirementInfo={} %GIDa_0e3e2a32_c8b7_428f_ab0c_0faebbbf5e76  Gain=32.174
  k5 : Gain  RequirementInfo={} %GIDa_be5380e6_e279_4fba_b4a2_cea2808c46f4  Gain=180/pi
  k6 : Gain  RequirementInfo={} %GIDa_bccc5425_7281_49cf_93c6_a752e7732049  Gain=2
  omegaSq : Product  RequirementInfo={} %GIDa_e5c95743_58d1_4d7b_8e0f_0d5dca474f7a  RndMeth=Zero
  omegaSq2 : Product  RequirementInfo={} %GIDa_907b30dd_aede_4316_9a8a_044ea704cef8  RndMeth=Zero
  HdgCmd : Outport  RequirementInfo={} %GIDa_7c7f0b37_435d_4e7c_952c_62c879fcb657
  HdgRteCmd : Outport  RequirementInfo={} %GIDa_0b79bbaa_a2da_4cb9_814f_266c555013e7  Port=2
  wires:
  Integrator1/1 -> Sum2/2, HdgCmd/1, HdgCmdScope/3  "HdgCmd"
  Vt/1 -> k2/1
  k2/1 -> Saturation/1  "VTfps"
  k/1 -> Saturation Dynamic1/3
  RollLimit/1 -> k3/1
  Sum3/1 -> Saturation Dynamic1/2  "eaccel"
  Saturation Dynamic1/1 -> VarLimIntegIC/3(In), HdgCmdScope/1  "LimAccel"
  k3/1 -> Trigonometric Function/1
  Trigonometric Function/1 -> k4/1
  k4/1 -> k5/1
  k5/1 -> Product3/1
  Product3/1 -> VarLimIntegIC/1(UpLim), k1/1  "RateLim"
  k1/1 -> VarLimIntegIC/2(LoLim)
  VarLimIntegIC/1(Out) -> Integrator1/1, HdgCmdScope/2, 2zetaOmega/1, HdgRteCmd/1  "LimRate"
  k6/1 -> 2zetaOmega/2
  2zetaOmega/1 -> Sum3/2
  init/1 -> VarLimIntegIC/5(IC)
  omegaSq/1 -> omegaSq2/1
  omegaSq2/1 -> Sum3/1
  Sum2/1 -> ANGL/1(in)  "epos"
  HdgCmdMCP/1 -> Logical Operator/1, Sum2/1, HdgCmdScope/4  "Cmd"
  ANGL/1(180) -> omegaSq2/2
  Logical Operator/1 -> VarLimIntegIC/4(Trig), Integrator1/2
  Saturation/1 -> Product1/2, Product2/2, Product3/2
  Heading/1 -> Integrator1/3
  Product2/1 -> Saturation Dynamic1/1, k/1
  Constant/1 -> Sum/1
  Constant1/1 -> Product1/1
  Product1/1 -> Sum/2
  Constant2/1 -> Product2/1
  Sum/1 -> k6/1, omegaSq/1, omegaSq/2  "omega"

== system ControlsWithAutopilot_Properties/Heading/Heading Control/VarLimIntegIC ==
  UpLim : Inport  RequirementInfo={} %GIDa_a52f7b7f_3cd2_4b84_aa46_8f49d190de5c
  LoLim : Inport  RequirementInfo={} %GIDa_14f49477_0466_41ac_a405_ff8b353df89c  Port=2
  In : Inport  RequirementInfo={} %GIDa_3e285f49_2930_4df4_81dd_a9b406bbe3bd  Port=3
  Trig : Inport  RequirementInfo={} %GIDa_a10733bc_08b5_4d2b_a4b2_d21b5a57b6cc  Port=4
  IC : Inport  RequirementInfo={} %GIDa_1f0c5f5f_64dd_4362_ac43_aa1a0320c078  Port=5
  Constant1 : Constant  RequirementInfo={} %GIDa_06ecceb0_a33e_4777_98b5_cbb205f23b1a  Value=0
  Constant2 : Constant  RequirementInfo={} %GIDa_450747a0_c4d7_4d05_b9cd_637cc0a6e70e  Value=0
  Constant3 : Constant  RequirementInfo={} %GIDa_2162f9e8_6490_497e_a11b_22bba3b34cf8  Value=0
  Integrator : DiscreteIntegrator  ExternalReset=level  InitialConditionSource=external  SampleTime=1.0  mask(DiscretizedDiscreteIntegrator){}
      mask init:
      | %zoh
  Logical Operator : Logic  RequirementInfo={} %GIDa_08f35c7f_9ec6_4cc6_9a1f_42b21408c66a  AllPortsSameDT=off
  Logical Operator1 : Logic  RequirementInfo={} %GIDa_78d08ac2_a159_4fb8_990a_70ef898240f1  AllPortsSameDT=off
  Logical Operator2 : Logic  RequirementInfo={} %GIDa_16203443_42bb_4de7_9e01_30a8f399b69b  Operator=OR  AllPortsSameDT=off
  Relational Operator : RelationalOperator  RequirementInfo={} %GIDa_fd2b09f2_7292_41cd_b490_47957a93b770  Operator=<=
  Relational Operator1 : RelationalOperator  RequirementInfo={} %GIDa_bc21e44d_a4ad_4459_a4e5_c40c404b3dbb
  Relational Operator2 : RelationalOperator  RequirementInfo={} %GIDa_257b199b_80e3_40b3_851a_c63ec13dd9de  Operator=>
  Relational Operator3 : RelationalOperator  RequirementInfo={} %GIDa_34126d1c_0a68_4b2a_a8f9_adf647778def  Operator=<
  Switch1 : Switch  RequirementInfo={} %GIDa_093ada51_26d0_4dd4_951b_93ea95402387  Threshold=0.5  SaturateOnIntegerOverflow=on  InputSameDT=on
  Switch2 : Switch  RequirementInfo={} %GIDa_ce0381f3_056e_496f_90b9_8ff8975dbd4b  Threshold=0.5  SaturateOnIntegerOverflow=on  InputSameDT=on
  Switch3 : Switch  RequirementInfo={} %GIDa_23ed59f4_3b4c_47cd_8936_54e05a064030  Threshold=0.5  SaturateOnIntegerOverflow=on  InputSameDT=on
  Out : Outport  RequirementInfo={} %GIDa_a2a80f39_47d8_4649_81f4_5246420c0c65
  wires:
  Relational Operator1/1 -> Logical Operator1/2, Switch2/2
  Switch1/1 -> Switch2/3, Relational Operator1/2
  LoLim/1 -> Relational Operator1/1, Switch2/1
  IC/1 -> Integrator/3
  Trig/1 -> Integrator/2
  Constant2/1 -> Relational Operator3/2
  Relational Operator3/1 -> Logical Operator1/1
  Logical Operator1/1 -> Logical Operator2/2
  Logical Operator/1 -> Logical Operator2/1
  Logical Operator2/1 -> Switch3/2
  Relational Operator2/1 -> Logical Operator/2
  Constant1/1 -> Relational Operator2/2
  In/1 -> Switch3/3, Relational Operator3/1, Relational Operator2/1
  Constant3/1 -> Switch3/1
  Switch3/1 -> Integrator/1
  Relational Operator/1 -> Logical Operator/1, Switch1/2
  Switch2/1 -> Out/1
  UpLim/1 -> Switch1/1, Relational Operator/1
  Integrator/1 -> Relational Operator/2, Switch1/3

== system ControlsWithAutopilot_Properties/Heading/Roll InnerLoop/Kcas_pp ==
  In : Inport
  CompInfEq2 : RelationalOperator  Operator=<=  InputSameDT=on
  CompInfEq3 : RelationalOperator  Operator=<=  InputSameDT=on
  CompInfEq4 : RelationalOperator  Operator=<=  InputSameDT=on
  CompSup1 : RelationalOperator  InputSameDT=on
  CompSup2 : RelationalOperator  Operator=>  InputSameDT=on
  CompSup3 : RelationalOperator  Operator=>  InputSameDT=on
  Data1 : Constant
  Data2 : Constant
  Data3 : Constant  Value=0.3
  Data4 : Constant  Value=0.3
  Idx1 : Constant  Value=0
  Idx2 : Constant  Value=120
  Idx3 : Constant  Value=350
  Idx4 : Constant  Value=500
  Interpolate1 : Subsystem
  Interpolate2 : Subsystem
  Interpolate3 : Subsystem
  Product1 : Product  Inputs=***  SaturateOnIntegerOverflow=on  RndMeth=Zero  OutDataTypeStr=Inherit: Same as first input
  Product2 : Product  Inputs=***  SaturateOnIntegerOverflow=on  RndMeth=Zero  OutDataTypeStr=Inherit: Same as first input
  Product3 : Product  Inputs=***  SaturateOnIntegerOverflow=on  RndMeth=Zero  OutDataTypeStr=Inherit: Same as first input
  Sum : Sum  Inputs=+++  SaturateOnIntegerOverflow=on  InputSameDT=on  OutDataTypeStr=Inherit: Same as first input
  Out : Outport
  wires:
  In/1 -> Interpolate1/1(InportIn), CompSup1/1, Interpolate2/1(InportIn), CompSup2/1, CompInfEq2/1, Interpolate3/1(InportIn), CompSup3/1, CompInfEq3/1, CompInfEq4/1
  Idx1/1 -> Interpolate1/2(InportIdx1), CompSup1/2
  Data1/1 -> Interpolate1/4(InportData1)
  Interpolate1/1(Out) -> Product1/1
  CompSup1/1 -> Product1/2
  CompInfEq2/1 -> Product1/3
  Product1/1 -> Sum/1
  Idx2/1 -> Interpolate2/2(InportIdx1), CompSup2/2, Interpolate1/3(InportIdx2), CompInfEq2/2
  Data2/1 -> Interpolate2/4(InportData1), Interpolate1/5(InportData2)
  Interpolate2/1(Out) -> Product2/1
  CompSup2/1 -> Product2/2
  CompInfEq3/1 -> Product2/3
  Product2/1 -> Sum/2
  Idx3/1 -> Interpolate3/2(InportIdx1), CompSup3/2, Interpolate2/3(InportIdx2), CompInfEq3/2
  Data3/1 -> Interpolate3/4(InportData1), Interpolate2/5(InportData2)
  Interpolate3/1(Out) -> Product3/1
  CompSup3/1 -> Product3/2
  CompInfEq4/1 -> Product3/3
  Product3/1 -> Sum/3
  Idx4/1 -> Interpolate3/3(InportIdx2), CompInfEq4/2
  Data4/1 -> Interpolate3/5(InportData2)
  Sum/1 -> Out/1

== system ControlsWithAutopilot_Properties/Longitudinal/Altitude Control/Variable  Rate Limit ==
  ratelim : Inport  RequirementInfo={} %GIDa_1ef85aab_f902_404e_a68b_00e57673dd3f
  input : Inport  RequirementInfo={} %GIDa_7ac59940_1fcc_4039_a5aa_a007950c590e  Port=2
  ICtrig : Inport  RequirementInfo={} %GIDa_9850dee7_08ca_49d5_88fb_399ee4ba203e  Port=3
  IC : Inport  RequirementInfo={} %GIDa_d80fe626_91fd_4f82_ad17_86aca6b3aee5  Port=4
  Gain : Gain  RequirementInfo={} %GIDa_55467e41_3bd6_44bf_9a44_6f78661bf8f0  Gain=20  SaturateOnIntegerOverflow=on  OutDataTypeStr=Inherit: Same as input  ParamDataTypeStr=Inherit: Same as input
  Gain1 : Gain  RequirementInfo={} %GIDa_0b7dd2e9_dfcf_42d3_8fb1_8c254e005ceb  Gain=-1  SaturateOnIntegerOverflow=on  OutDataTypeStr=Inherit: Same as input  ParamDataTypeStr=Inherit: Same as input
  Integrator : DiscreteIntegrator  ExternalReset=level  InitialConditionSource=external  SampleTime=1.0  mask(DiscretizedDiscreteIntegrator){}
      mask init:
      | %zoh
  Sum2 : Sum  RequirementInfo={} %GIDa_de9ff84b_54f5_48bc_9ef3_874415208380  Inputs=|+-  SaturateOnIntegerOverflow=on
  Variable Limit Saturation : Subsystem  RequirementInfo={} %GIDa_42540829_63e9_4d83_adf5_d7c684208c2d
  output : Outport  RequirementInfo={} %GIDa_74eb2916_410f_4b2d_afdf_0d476e7e03b7
  wires:
  Sum2/1 -> Gain/1
  Gain/1 -> Variable Limit Saturation/2(SigIn)
  ratelim/1 -> Gain1/1, Variable Limit Saturation/1(up_lim)
  Gain1/1 -> Variable Limit Saturation/3(Lo_lim)
  Variable Limit Saturation/1(Out1) -> Integrator/1
  Integrator/1 -> Sum2/2, output/1
  input/1 -> Sum2/1
  ICtrig/1 -> Integrator/2
  IC/1 -> Integrator/3

== system ControlsWithAutopilot_Properties/Longitudinal/Altitude Control/Variable Limit Saturation ==
  up_lim : Inport  RequirementInfo={} %GIDa_a8c5a358_1294_4ae6_a63f_3940fe218386
  SigIn : Inport  RequirementInfo={} %GIDa_062a0af8_40f0_4204_856b_8e0aded8de05  Port=2
  Lo_lim : Inport  RequirementInfo={} %GIDa_6793747b_c094_4bd9_a5cb_839f8eb54e21  Port=3
  Enforce low lim : MinMax  RequirementInfo={} %GIDa_e93f4b97_2f8b_4f52_84c9_3cb68ddf7e16  Function=max  Inputs=2
  Enforce up lim : MinMax  RequirementInfo={} %GIDa_c018e6ad_c664_4361_a96c_d990e2efb7d8  Inputs=2
  Out1 : Outport  RequirementInfo={} %GIDa_0d7a9d35_dde5_41a4_a708_f2de214bfa54
  wires:
  Lo_lim/1 -> Enforce low lim/1
  SigIn/1 -> Enforce low lim/2
  Enforce low lim/1 -> Enforce up lim/1
  up_lim/1 -> Enforce up lim/2
  Enforce up lim/1 -> Out1/1
